simulink model "cdip_swing_up2_sim"  (R2013a)
settings: Solver=ode4  StartTime=0.0  StopTime=16  FixedStep=0.001  RelTol=1e-3
values from neighbouring files (symbols this model uses):
  B = [ zeros(2,1) ... (first row only)    [p2c323_Sliding_Mode_Control.m]
  delta = 0    [p2c323_ex1_cdip_swing_up.m]    (also in p2c323_ex1_cdip_swing_up_custum.m)
  dtheta_0 = 0    [p2c323_ex1_cdip_swing_up.m]    (also in p2c323_ex1_cdip_swing_up_custum.m)
  dz_0 = 0    [p2c323_ex1_cdip_swing_up.m]    (also in p2c323_ex1_cdip_swing_up_custum.m)
  K1 = 0.8    [p2c323_ex1_cdip_swing_up.m]    (also in p2c323_ex1_cdip_swing_up_custum.m)
  K2 = 30    [p2c323_ex1_cdip_swing_up.m]    (also in p2c323_ex1_cdip_swing_up_custum.m)
  S = ( [Ab12'*P+Qb12'  Qb22]*T )'    [p2c323_Sliding_Mode_Control.m]
  switch_angle = pi/4    (= 0.785398163397)    [p2c323_ex1_cdip_swing_up.m]    (also in p2c323_ex1_cdip_swing_up_custum.m)
  theta_0 = pi + 0.001    (= 3.14259265359)    [p2c323_ex1_cdip_swing_up.m]    (also in p2c323_ex1_cdip_swing_up_custum.m)
  z_0 = 0.1    [p2c323_ex1_cdip_swing_up.m]    (also in p2c323_ex1_cdip_swing_up_custum.m)
undefined symbols (not defined in the file or in its folder): ac, bc, g, Jp, lp, mp, mup
settings Model: Creator=kawata  LastModifiedBy=kawata

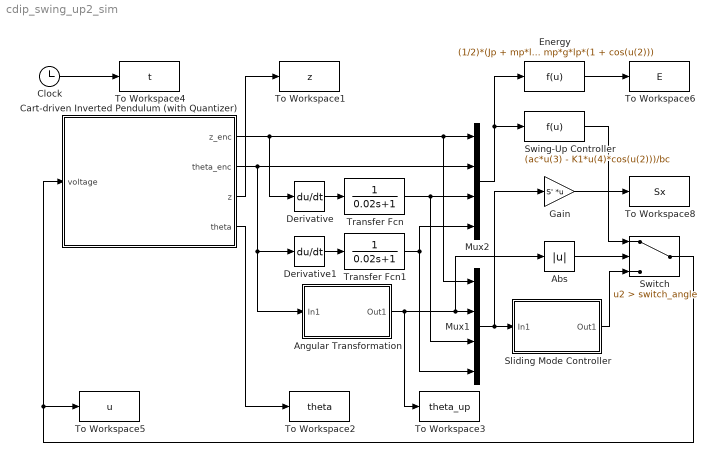
== system cdip_swing_up2_sim ==
  Abs : Abs
  Angular Transformation : Subsystem
  Cart-driven Inverted Pendulum (with Quantizer) : Subsystem
      mask Display: image(imread('cdip_photo.jpg'),'center')
  Clock : Clock
  Derivative : Derivative
  Derivative1 : Derivative
  Energy : Fcn  Expr=(1/2)*(Jp + mp*lp^2)*u(4)^2 + mp*g*lp*(1 + cos(u(2)))
  Gain : Gain  Gain=S'  Multiplication=Matrix(K*u)  SaturateOnIntegerOverflow=on  OutDataTypeStr=Inherit: Same as input  ParamDataTypeStr=Inherit: Same as input
  Mux1 : Mux
  Mux2 : Mux
  Sliding Mode Controller : Subsystem
  Swing-Up Controller : Fcn  Expr=(ac*u(3) - K1*u(4)*cos(u(2)))/bc
  Switch : Switch  Criteria=u2 > Threshold  Threshold=switch_angle
  To Workspace1 : ToWorkspace  VariableName=z  SampleTime=-1
  To Workspace2 : ToWorkspace  VariableName=theta  SampleTime=-1
  To Workspace3 : ToWorkspace  VariableName=theta_up  SampleTime=-1
  To Workspace4 : ToWorkspace  VariableName=t  SampleTime=-1
  To Workspace5 : ToWorkspace  VariableName=u  SampleTime=-1
  To Workspace6 : ToWorkspace  VariableName=E  SampleTime=-1
  To Workspace8 : ToWorkspace  VariableName=Sx  SampleTime=-1
  Transfer Fcn : TransferFcn  Denominator=[0.02 1]
  Transfer Fcn1 : TransferFcn  Denominator=[0.02 1]
  wires:
  Cart-driven Inverted Pendulum (with Quantizer)/1(z_enc) -> Mux2/1, Mux1/1, Derivative/1
  Transfer Fcn/1 -> Mux2/3, Mux1/3
  Clock/1 -> To Workspace4/1
  Swing-Up Controller/1 -> Switch/1
  Switch/1 -> Cart-driven Inverted Pendulum (with Quantizer)/1(voltage), To Workspace5/1
  Energy/1 -> To Workspace6/1
  Cart-driven Inverted Pendulum (with Quantizer)/2(theta_enc) -> Mux2/2, Angular Transformation/1(In1), Derivative1/1
  Angular Transformation/1(Out1) -> Mux1/2, Abs/1, To Workspace3/1
  Abs/1 -> Switch/2
  Gain/1 -> To Workspace8/1
  Sliding Mode Controller/1(Out1) -> Switch/3
  Derivative/1 -> Transfer Fcn/1
  Derivative1/1 -> Transfer Fcn1/1
  Transfer Fcn1/1 -> Mux2/4, Mux1/4
  Cart-driven Inverted Pendulum (with Quantizer)/3(z) -> To Workspace1/1
  Cart-driven Inverted Pendulum (with Quantizer)/4(theta) -> To Workspace2/1
  Mux1/1 -> Sliding Mode Controller/1(In1), Gain/1
  Mux2/1 -> Swing-Up Controller/1, Energy/1

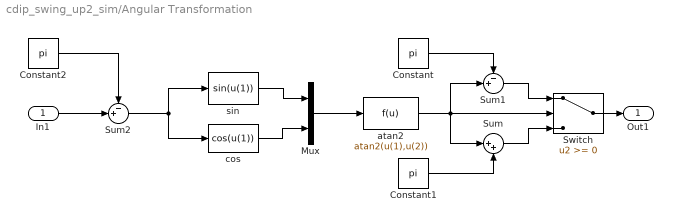
== system cdip_swing_up2_sim/Angular Transformation ==
  In1 : Inport
  Constant : Constant  Value=pi
  Constant1 : Constant  Value=pi
  Constant2 : Constant  Value=pi
  Mux : Mux  Inputs=2
  Sum : Sum  Inputs=|++  SaturateOnIntegerOverflow=on  InputSameDT=on  OutDataTypeStr=Inherit: Same as first input
  Sum1 : Sum  Inputs=-+|  SaturateOnIntegerOverflow=on  InputSameDT=on  OutDataTypeStr=Inherit: Same as first input
  Sum2 : Sum  Inputs=-+|  SaturateOnIntegerOverflow=on  InputSameDT=on  OutDataTypeStr=Inherit: Same as first input
  Switch : Switch
  atan2 : Fcn  Expr=atan2(u(1),u(2))
  cos : Fcn  Expr=cos(u(1))
  sin : Fcn  Expr=sin(u(1))
  Out1 : Outport
  wires:
  Mux/1 -> atan2/1
  cos/1 -> Mux/2
  sin/1 -> Mux/1
  atan2/1 -> Sum/1, Switch/2, Sum1/2
  Sum1/1 -> Switch/1
  Constant1/1 -> Sum/2
  Sum/1 -> Switch/3
  Constant/1 -> Sum1/1
  Switch/1 -> Out1/1
  Constant2/1 -> Sum2/1
  In1/1 -> Sum2/2
  Sum2/1 -> cos/1, sin/1

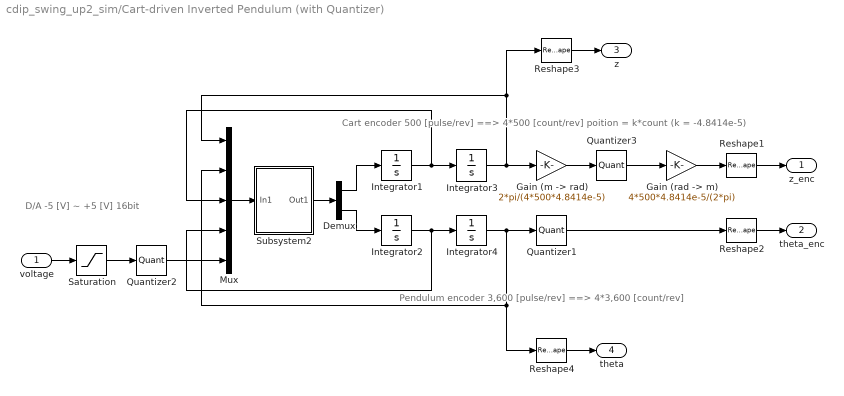
== system cdip_swing_up2_sim/Cart-driven Inverted Pendulum (with Quantizer) ==
  note: Cart encoder
      |   500 [pulse/rev]  ==> 4*500 [count/rev]
      |   poition = k*count  (k = -4.8414e-5)
  note: D/A
      |   -5 [V] ~ +5 [V]
      |  16bit
  note: Pendulum encoder
      |   3,600 [pulse/rev]  ==> 4*3,600 [count/rev]
  voltage : Inport
  Demux : Demux  Outputs=2
  "Gain (m -> rad)" : Gain  Gain=2*pi/(4*500*4.8414e-5)  SaturateOnIntegerOverflow=on  OutDataTypeStr=Inherit: Same as input  ParamDataTypeStr=Inherit: Same as input
  "Gain (rad -> m)" : Gain  Gain=4*500*4.8414e-5/(2*pi)  SaturateOnIntegerOverflow=on  OutDataTypeStr=Inherit: Same as input  ParamDataTypeStr=Inherit: Same as input
  Integrator1 : Integrator  InitialCondition=dz_0
  Integrator2 : Integrator  InitialCondition=dtheta_0
  Integrator3 : Integrator  InitialCondition=z_0
  Integrator4 : Integrator  InitialCondition=theta_0
  Mux : Mux  Inputs=5
  Quantizer1 : Quantizer  QuantizationInterval=2*pi/(4*3600)
  Quantizer2 : Quantizer  QuantizationInterval=10/2^(16)
  Quantizer3 : Quantizer  QuantizationInterval=2*pi/(4*500)
  Reshape{1..4} (4 alike) : Reshape
  Saturation : Saturate  UpperLimit=5  LowerLimit=-5
  Subsystem2 : Subsystem
  z_enc : Outport
  theta_enc : Outport  Port=2
  z : Outport  Port=3
  theta : Outport  Port=4
  wires:
  Reshape4/1 -> theta/1
  Reshape3/1 -> z/1
  Saturation/1 -> Quantizer2/1
  Quantizer2/1 -> Mux/5
  Quantizer1/1 -> Reshape2/1
  Subsystem2/1(Out1) -> Demux/1
  Mux/1 -> Subsystem2/1(In1)
  Demux/1 -> Integrator1/1
  Demux/2 -> Integrator2/1
  Integrator1/1 -> Mux/3, Integrator3/1
  Integrator2/1 -> Mux/4, Integrator4/1
  Integrator3/1 -> Reshape3/1, Mux/1, "Gain (m -> rad)"/1
  Integrator4/1 -> Reshape4/1, Mux/2, Quantizer1/1
  voltage/1 -> Saturation/1
  "Gain (m -> rad)"/1 -> Quantizer3/1
  Quantizer3/1 -> "Gain (rad -> m)"/1
  "Gain (rad -> m)"/1 -> Reshape1/1
  Reshape1/1 -> z_enc/1
  Reshape2/1 -> theta_enc/1

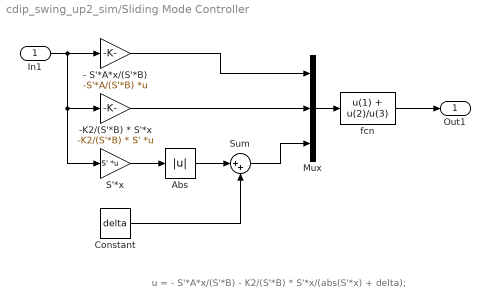
== system cdip_swing_up2_sim/Sliding Mode Controller ==
  note: u = - S'*A*x/(S'*B) - K2/(S'*B) * S'*x/(abs(S'*x) + delta);
  In1 : Inport
  - S'*A*x/(S'*B) : Gain  Gain=-S'*A/(S'*B)  Multiplication=Matrix(K*u)  SaturateOnIntegerOverflow=on  OutDataTypeStr=Inherit: Same as input  ParamDataTypeStr=Inherit: Same as input
  -K2/(S'*B) * S'*x : Gain  Gain=-K2/(S'*B) * S'  Multiplication=Matrix(K*u)  SaturateOnIntegerOverflow=on  OutDataTypeStr=Inherit: Same as input  ParamDataTypeStr=Inherit: Same as input
  Abs : Abs
  Constant : Constant  Value=delta
  Mux : Mux  Inputs=3
  S'*x : Gain  Gain=S'  Multiplication=Matrix(K*u)  SaturateOnIntegerOverflow=on  OutDataTypeStr=Inherit: Same as input  ParamDataTypeStr=Inherit: Same as input
  Sum : Sum  Inputs=|++  SaturateOnIntegerOverflow=on  InputSameDT=on  OutDataTypeStr=Inherit: Same as first input
  fcn : Fcn  Expr=u(1) + u(2)/u(3)
  Out1 : Outport
  wires:
  In1/1 -> S'*x/1, -K2/(S'*B) * S'*x/1, - S'*A*x/(S'*B)/1
  Constant/1 -> Sum/2
  S'*x/1 -> Abs/1
  Abs/1 -> Sum/1
  Mux/1 -> fcn/1
  - S'*A*x/(S'*B)/1 -> Mux/1
  -K2/(S'*B) * S'*x/1 -> Mux/2
  Sum/1 -> Mux/3
  fcn/1 -> Out1/1

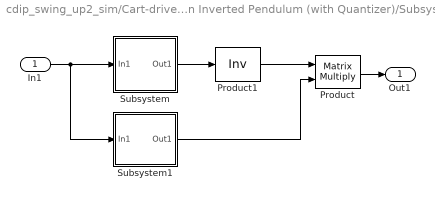
== system cdip_swing_up2_sim/Cart-driven Inverted Pendulum (with Quantizer)/Subsystem2 ==
  In1 : Inport
  Product : Product  Multiplication=Matrix(*)  SaturateOnIntegerOverflow=on  InputSameDT=on  OutDataTypeStr=Inherit: Same as first input
  Product1 : Product  Inputs=/  Multiplication=Matrix(*)  SaturateOnIntegerOverflow=on  InputSameDT=on  OutDataTypeStr=Inherit: Same as first input
  Subsystem : Subsystem
  Subsystem1 : Subsystem
  Out1 : Outport
  wires:
  Subsystem/1(Out1) -> Product1/1
  Product1/1 -> Product/1
  Subsystem1/1(Out1) -> Product/2
  In1/1 -> Subsystem/1(In1), Subsystem1/1(In1)
  Product/1 -> Out1/1

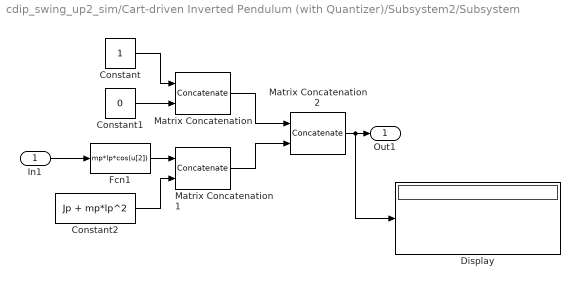
== system cdip_swing_up2_sim/Cart-driven Inverted Pendulum (with Quantizer)/Subsystem2/Subsystem ==
  In1 : Inport
  Constant : Constant
  Constant1 : Constant  Value=0
  Constant2 : Constant  Value=Jp + mp*lp^2
  Display : Display
  Fcn1 : Fcn  Expr=mp*lp*cos(u[2])
  Matrix Concatenation : Concatenate  Mode=Multidimensional array  ConcatenateDimension=2
  Matrix Concatenation1 : Concatenate  Mode=Multidimensional array  ConcatenateDimension=2
  Matrix Concatenation2 : Concatenate  Mode=Multidimensional array
  Out1 : Outport
  wires:
  Constant2/1 -> Matrix Concatenation1/2
  Fcn1/1 -> Matrix Concatenation1/1
  In1/1 -> Fcn1/1
  Matrix Concatenation/1 -> Matrix Concatenation2/1
  Matrix Concatenation1/1 -> Matrix Concatenation2/2
  Matrix Concatenation2/1 -> Display/1, Out1/1
  Constant/1 -> Matrix Concatenation/1
  Constant1/1 -> Matrix Concatenation/2

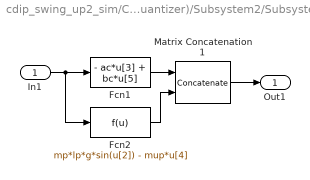
== system cdip_swing_up2_sim/Cart-driven Inverted Pendulum (with Quantizer)/Subsystem2/Subsystem1 ==
  In1 : Inport
  Fcn1 : Fcn  Expr=- ac*u[3] + bc*u[5]
  Fcn2 : Fcn  Expr=mp*lp*g*sin(u[2]) - mup*u[4]
  Matrix Concatenation1 : Concatenate  Mode=Multidimensional array
  Out1 : Outport
  wires:
  Fcn2/1 -> Matrix Concatenation1/2
  Fcn1/1 -> Matrix Concatenation1/1
  In1/1 -> Fcn2/1, Fcn1/1
  Matrix Concatenation1/1 -> Out1/1
